simulink model "COMPONENT_MDL_Lag_QUAD_and_PEND_with_Ab"  (R2020b)
settings: Solver=ode23t  StartTime=0.0  StopTime=200  FixedStep=0.001  RelTol=1e-5  EnableMultiTasking=on
undefined symbols (not defined in the file or in its folder): P_pend, P_rot, P_veh_no_props
(part 1 of 12)
settings Model: Creator=bhorton  LastModifiedBy=bhorton
settings DataIOCC: SaveOutput=off  SignalLogging=off  DSMLogging=off  VisualizeSimOutput=off  SaveTime=off  ReturnWorkspaceOutputs=off
settings OptimizationCC: LifeSpan=inf
settings DebuggingCC: AllowSymbolicDim=off  PregeneratedLibrarySubsystemCodeDiagnostic=none  SFUnexpectedBacktrackingDiag=warning  SFNoUnconditionalDefaultTransitionDiag=warning  SFExecutionAtInitializationDiag=none  ArithmeticOperatorsInVariantConditions=warning
settings ModelReferenceCC: PropagateSignalLabelsOutOfModel=off
settings SFSimCC: SimUseLocalCustomCode=off  CustomCodeUndefinedFunction=UseInterfaceOnly
settings RTWCC: RTWUseLocalCustomCode=off
settings CodeAppCC: StateflowObjectComments=on
settings GRTTargetCC: TargetLangStandard=C89/C90 (ANSI)
settings ConfigComp: CovMetricSettings=dw  CovSaveCumulativeToWorkspaceVar=on  CovSaveSingleToWorkspaceVar=on  CovExternalEMLEnable=off
settings SimscapeCC: SimscapeNormalizeSystem=off

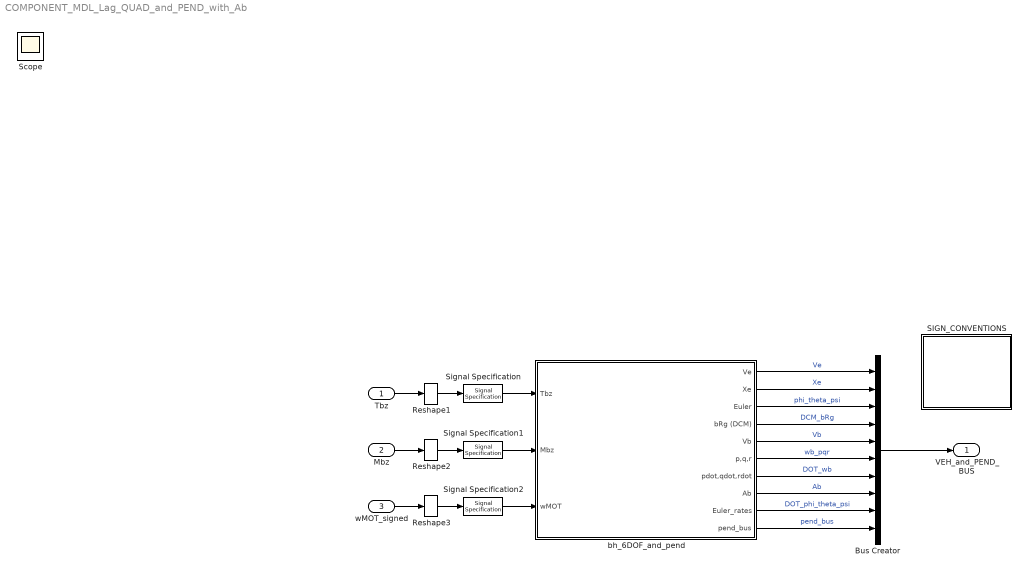
== system COMPONENT_MDL_Lag_QUAD_and_PEND_with_Ab ==
  Tbz : Inport
  Mbz : Inport  Port=2
  wMOT_signed : Inport  Port=3
  Bus Creator : BusCreator  Inputs=10
  Reshape1 : Reshape  OutputDimensionality=Column vector (2-D)
  Reshape2 : Reshape  OutputDimensionality=Column vector (2-D)
  Reshape3 : Reshape  OutputDimensionality=Column vector (2-D)
  SIGN_CONVENTIONS : Subsystem
  Signal Specification : SignalSpecification  Dimensions=[4,1]
  Signal Specification1 : SignalSpecification  Dimensions=[4,1]
  Signal Specification2 : SignalSpecification  Dimensions=[4,1]
  bh_6DOF_and_pend : Subsystem  mask(bh_6DOF EoM (Body Axis)){air_inertia_0=P_veh_no_props.I, air_mass_0=P_veh_no_props.mass, xme_0=P_veh_no_props.Xe_init, Vm_0=P_veh_no_props.Vb_init, pm_0=P_veh_no_props.wb_init, eul_0=P_veh_no_props.eul_init, prop_Imat=P_rot.I, prop_mass=P_rot.mass, prop_CG_L=P_veh_no_props.L_CG_to_mot, prop_CG_H=P_veh_no_props.H_CG_to_mot, g_const=9.80665, I_pend=P_pend.I, m_pend=P_pend.mass, L_pend_XYZ=P_pend.L_xyz, T_pend_XYZ=P_pend.T_xyz, eul_0_pend=P_pend.eul_loc_vec}
      mask prompts: air_inertia_0 "Airframe Inertia, [kg.m^2]"; air_mass_0 "Airframe Mass, [kg]"; xme_0 "Initial position in inertial axes [Xe,Ye,Ze], [m]"; Vm_0 "Initial velocity in body axes [U,v,w], [m/sec]"; pm_0 "Initial body rotation rates [p,q,r], [rad/sec]"; eul_0 "Initial Euler orientation [yaw, pitch, roll], [rad]"; prop_Imat "Propeller Assembly Inertia [kg*m^2]"; prop_mass "Propeller Assembly Mass [kg]"; prop_CG_L "Airframe CG to Prop CG distance - L [m]"; prop_CG_H "Airframe CG to Prop CG distance - H [m]"; g_const "Gravity constant [m/sec^2]"; I_pend "Inertia of Pendulum through it's CoM [kg.m^2]"; m_pend "Mass of pendulum [kg]"; L_pend_XYZ "Lengths of Pendulum (X,Y,Z)  [m]"; T_pend_XYZ "Position of Spherical joint T(X,Y,Z) [m]"; eul_0_pend "Initial Euler orientation [yaw, pitch, roll], [rad]"
      mask DialogControl DescTextVar Prompt: Implementation of a 6-DOF rigid body equations of motion.
      mask DialogControl Control16 Prompt: Euler angles are used to describe angular pose.
      mask DialogControl Container4 Prompt: Airframe
      mask DialogControl Control11 Prompt: ATTENTION:  note the order of the angles in the list above.
      mask DialogControl Control12 Prompt: This is DIFFERENT to the order used in the Aerospace blockset.
      mask DialogControl Container19 Prompt: Propeller
      mask DialogControl Container13 Prompt: ENVIRONMENT
      mask DialogControl Control42 Prompt: NOTE:  the Gravity constant should be a POSITIVE number, eg: 9.81
      mask DialogControl Container14 Prompt: Pendulum
      mask DialogControl Control50 Prompt: Position of Spherical joint relative to airframe CoM:
      mask DialogControl Control41 Prompt: Define the Euler angles of {P}-frame relative to {V}-frame.  The rotation
      mask DialogControl Control45 Prompt: sequence is Z-Y-X  as [Phi,Theta,Psi]
      mask DialogControl Container20 Prompt: Geometry
      mask DialogControl Container21 Prompt: Axes
      mask DialogControl Container6 Prompt: DOC
      mask DialogControl Control6 Prompt: In this EULER angle implementation we define the
      mask DialogControl Control7 Prompt: following sequence that rotates a G-frame
      mask DialogControl Control8 Prompt: into a B-frame:
      mask DialogControl Control9_copy Prompt: 1.)  R1Z  : a local rotation about the Z axis by phi, (YAW)
      mask DialogControl Control9_copy_copy Prompt: 2.)  R2Y  : a local rotation about the Y axis by theta, (PITCH)
      mask DialogControl Control17 Prompt: 3.)  R3X  : a local rotation about the X axis by psi, (ROLL)
      mask DialogControl Container16 Prompt: PASSIVE rotation sequence
      mask DialogControl Control22 Prompt: The co-ordinate transformation that converts the components of a
      mask DialogControl Control23 Prompt: G-frame vector into its components in the B-frame, is:
      mask DialogControl Control24 Prompt: vb = pR3X(psi) * pR2Y(theta) * pR1Z(phi) * vg
      mask DialogControl Control25 Prompt: vb = bRg * vg
      mask DialogControl Control53 Prompt: You can READ more about PASSIVE rotations, HERE.
      mask DialogControl Control53 Callback: winopen('CONCEPT_PASSIVE_rotations.pdf')
      mask DialogControl Container22 Prompt: ACTIVE rotation sequence
      mask DialogControl Control26 Prompt: To actively reposition (ie: rotate) a B-frame that is initially coincident
      mask DialogControl Control27 Prompt: with the inertial G-frame, into a new pose, we would:
      mask DialogControl Control28 Prompt: vg = inv(pR1Z(phi)) * inv(pR2Y(theta)) * inv(pR3X(psi)) * vb
      mask DialogControl Control30 Prompt: If we define:    aR( ) == inv( pR()  ),  then we can write the above as:
      mask DialogControl Control32 Prompt: vg = aR1Z(phi) * aR2Y(theta) * aR3(psi) * vb
      mask DialogControl Control40 Prompt: You can READ more about ACTIVE rotations, HERE.
      mask DialogControl Control40 Callback: winopen('CONCEPT_ACTIVE_rotations.pdf')
      mask Display:
      | port_label('input',1,'{{Tbz_{mot}} (N)}','texmode','on');
      | port_label('input',2,'{{Mbz_{mot}} (N-m)}','texmode','on');
      | port_label('input',3,'{{\omega_{mot}} (rad/sec)}','texmode','on');
      | port_label('output',1,'{V_e (m/s)}','texmode','on');
      | port_label('output',2,'{X_e (m)}','texmode','on');
      | port_label('output',3,'{\Phi_{Z1} \theta_{Y2} \Psi_{X3} (rad)}','texmode','on');
      | port_label('output',4,'{DCM bRg }','texmode','on');
      | port_label('output',5,'{V_b (m/s)}','texmode','on');
      | port_label('output',6,'{{\omega_b (rad/s)}}','texmode','on');
      | port_label('output',7,'{{d\omega_b/dt}}','texmode','on');
      | port_label('output',8,'{A_b (m/s^2)}','texmode','on');
      | port_label('output',9,'{d\Phi_{Z1} d\theta_{Y2} d\Psi_{X3} (rad/sec)}','texmode','on');
      | 
      | %text(0.5,0.7248,'Simscape \nBody\nEuler Angles \n\n\n\n\n PENDULUM','horizontalAlignment','center')
      | %text(0.5,0.3112,'Fixed\nMass','horizontalAlignment','center')
      | %image(imread('bh_LAG_EQN.JPG'),[0.27, 0.25,0.5,0.35])
      | 
      | text(0.5,0.7248,'Quad\n+ PENDULUM','horizontalAlignment','center')
      | %text(0.5,0.3112,'Fixed\nMass','horizontalAlignment','center')
      | image(imread('bh_LAG_EQN.JPG'),[0.27, 0.25,0.5,0.35])
  VEH_and_PEND_BUS : Outport  OutDataTypeStr=Bus: VEH_AND_PEND_BUS  VectorParamsAs1DForOutWhenUnconnected=off
  Scope : Scope
  wires:
  wMOT_signed/1 -> Reshape3/1
  Tbz/1 -> Reshape1/1
  bh_6DOF_and_pend/6(p,q,r) -> Bus Creator/6  "wb_pqr"
  Bus Creator/1 -> VEH_and_PEND_BUS/1
  bh_6DOF_and_pend/7(pdot,qdot,rdot) -> Bus Creator/7  "DOT_wb"
  Reshape1/1 -> Signal Specification/1
  bh_6DOF_and_pend/1(Ve) -> Bus Creator/1  "Ve"
  Signal Specification2/1 -> bh_6DOF_and_pend/3(wMOT)
  Signal Specification/1 -> bh_6DOF_and_pend/1(Tbz)
  bh_6DOF_and_pend/9(Euler_rates) -> Bus Creator/9  "DOT_phi_theta_psi"
  bh_6DOF_and_pend/2(Xe) -> Bus Creator/2  "Xe"
  bh_6DOF_and_pend/8(Ab) -> Bus Creator/8  "Ab"
  Reshape3/1 -> Signal Specification2/1
  Reshape2/1 -> Signal Specification1/1
  bh_6DOF_and_pend/3(Euler) -> Bus Creator/3  "phi_theta_psi"
  Signal Specification1/1 -> bh_6DOF_and_pend/2(Mbz)
  bh_6DOF_and_pend/4(bRg (DCM)) -> Bus Creator/4  "DCM_bRg"
  bh_6DOF_and_pend/5(Vb) -> Bus Creator/5  "Vb"
  Mbz/1 -> Reshape2/1
  bh_6DOF_and_pend/10(pend_bus) -> Bus Creator/10  "pend_bus"

== system COMPONENT_MDL_Lag_QUAD_and_PEND_with_Ab/SIGN_CONVENTIONS ==

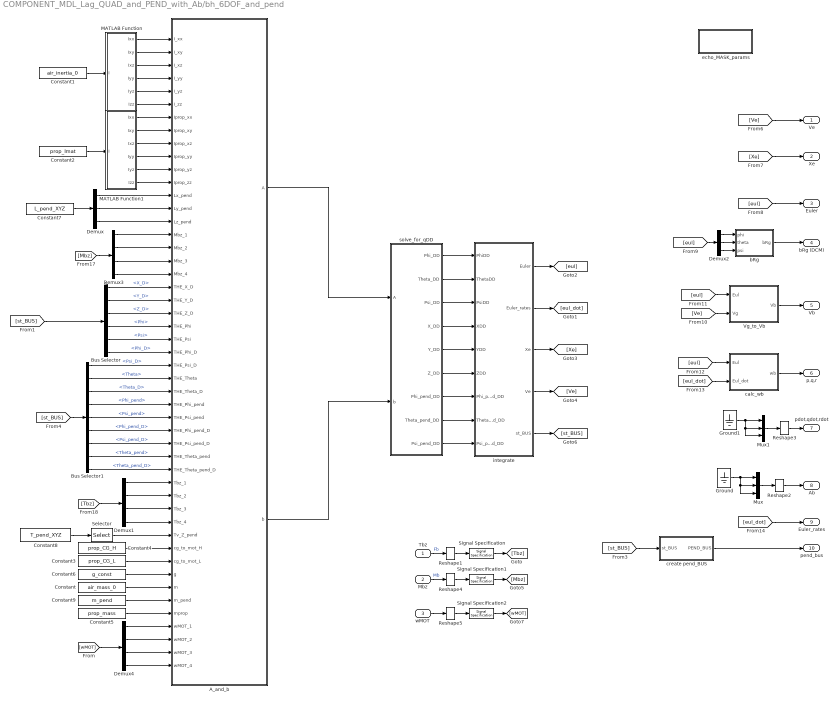
== system COMPONENT_MDL_Lag_QUAD_and_PEND_with_Ab/bh_6DOF_and_pend ==
  Tbz : Inport
  Mbz : Inport  Port=2
  wMOT : Inport  Port=3
  A_and_b : MATLAB Function  TreatAsAtomicUnit=on
  Bus Selector : BusSelector  OutputSignals=Vel_list.X_D,Vel_list.Y_D,Vel_list.Z_D,Pos_list.Phi,Pos_list.Psi,Vel_list.Phi_D
  Bus Selector1 : BusSelector  OutputSignals=Vel_list.Psi_D,Pos_list.Theta,Vel_list.Theta_D,Pos_list.Phi_pend,Pos_list.Psi_pend,Vel_list.Phi_pend_D,Vel_list.Psi_pend_D,Pos_list.Theta_pend,Vel_list.Theta_pend_D
  Constant : Constant  Value=air_mass_0  OutDataTypeStr=Inherit: Inherit via back propagation
  Constant1 : Constant  Value=air_inertia_0  OutDataTypeStr=Inherit: Inherit via back propagation
  Constant2 : Constant  Value=prop_Imat  OutDataTypeStr=Inherit: Inherit via back propagation
  Constant3 : Constant  Value=prop_CG_L  OutDataTypeStr=Inherit: Inherit via back propagation
  Constant4 : Constant  Value=prop_CG_H  OutDataTypeStr=Inherit: Inherit via back propagation
  Constant5 : Constant  Value=prop_mass  OutDataTypeStr=Inherit: Inherit via back propagation
  Constant6 : Constant  Value=g_const  OutDataTypeStr=Inherit: Inherit via back propagation
  Constant7 : Constant  Value=L_pend_XYZ  OutDataTypeStr=Inherit: Inherit via back propagation
  Constant8 : Constant  Value=T_pend_XYZ
  Constant9 : Constant  Value=m_pend  OutDataTypeStr=Inherit: Inherit via back propagation
  Demux : Demux  Outputs=3
  Demux1 : Demux
  Demux2 : Demux  Outputs=3
  Demux3 : Demux
  Demux4 : Demux
  Ground : Ground
  Ground1 : Ground
  MATLAB Function : MATLAB Function  TreatAsAtomicUnit=on
  MATLAB Function1 : MATLAB Function  TreatAsAtomicUnit=on
  Mux : Mux  Inputs=3
  Mux1 : Mux  Inputs=3
  Reshape{1..5} (5 alike) : Reshape  OutputDimensionality=Column vector (2-D)
  Selector : Selector  InputPortWidth=3  IndexOptions=Index vector (dialog)  Indices=3  OutputSizes=1
  Signal Specification : SignalSpecification  Dimensions=[4,1]
  Signal Specification1 : SignalSpecification  Dimensions=[4,1]
  Signal Specification2 : SignalSpecification  Dimensions=[4,1]
  Vg_to_Vb : Subsystem
  bRg : MATLAB Function  TreatAsAtomicUnit=on
  calc_wb : Subsystem
  create pend_BUS : Subsystem
  echo_MASK_params : Subsystem
  integrate : Subsystem
  solve_for_qDD : Subsystem
  Ve : Outport  VectorParamsAs1DForOutWhenUnconnected=off
  Xe : Outport  Port=2  VectorParamsAs1DForOutWhenUnconnected=off
  Euler : Outport  Port=3  VectorParamsAs1DForOutWhenUnconnected=off
  bRg (DCM) : Outport  Port=4  VectorParamsAs1DForOutWhenUnconnected=off
  Vb : Outport  Port=5  VectorParamsAs1DForOutWhenUnconnected=off
  p,q,r : Outport  Port=6  VectorParamsAs1DForOutWhenUnconnected=off
  pdot,qdot,rdot : Outport  Port=7  VectorParamsAs1DForOutWhenUnconnected=off
  Ab : Outport  Port=8  VectorParamsAs1DForOutWhenUnconnected=off
  Euler_rates : Outport  Port=9  VectorParamsAs1DForOutWhenUnconnected=off
  pend_bus : Outport  Port=10  VectorParamsAs1DForOutWhenUnconnected=off
  wires:
  Mux1/1 -> Reshape3/1
  MATLAB Function/5(Iyz) -> A_and_b/5(I_yz)
  Demux2/1 -> bRg/1(phi)
  Demux4/3 -> A_and_b/48(wMOT_3)
  Demux3/1 -> A_and_b/16(Mbz_1)
  [Xe] -> Xe/1
  MATLAB Function1/6(Izz) -> A_and_b/12(Iprop_zz)
  Tbz/1 -> Reshape1/1  "Fb"
  integrate/5(st_BUS) -> [st_BUS]
  Constant5/1 -> A_and_b/45(mprop)
  [Ve] -> Ve/1
  Ground/1 -> Mux/2, Mux/3, Mux/1
  Reshape3/1 -> pdot,qdot,rdot/1
  MATLAB Function1/2(Ixy) -> A_and_b/8(Iprop_xy)
  MATLAB Function/3(Ixz) -> A_and_b/3(I_xz)
  calc_wb/1(wb) -> p,q,r/1
  integrate/4(Ve) -> [Ve]
  Demux4/2 -> A_and_b/47(wMOT_2)
  Demux3/2 -> A_and_b/17(Mbz_2)
  [eul] -> Vg_to_Vb/1(Eul)
  Demux1/2 -> A_and_b/36(Tbz_2)
  [st_BUS] -> Bus Selector/1
  [Ve] -> Vg_to_Vb/2(Vg)
  Reshape4/1 -> Signal Specification1/1
  Demux1/1 -> A_and_b/35(Tbz_1)
  [eul] -> calc_wb/1(Eul)
  solve_for_qDD/5(Y_DD) -> integrate/5(YDD)
  MATLAB Function1/3(Ixz) -> A_and_b/9(Iprop_xz)
  Demux3/4 -> A_and_b/19(Mbz_4)
  integrate/1(Euler) -> [eul]
  [eul_dot] -> Euler_rates/1
  Demux2/3 -> bRg/3(psi)
  Constant/1 -> A_and_b/43(m)
  solve_for_qDD/6(Z_DD) -> integrate/6(ZDD)
  [Tbz] -> Demux1/1
  Mux/1 -> Reshape2/1
  solve_for_qDD/3(Psi_DD) -> integrate/3(PsiDD)
  Demux1/4 -> A_and_b/38(Tbz_4)
  MATLAB Function/2(Ixy) -> A_and_b/2(I_xy)
  Signal Specification/1 -> [Tbz]
  [eul_dot] -> calc_wb/2(Eul_dot)
  Demux4/1 -> A_and_b/46(wMOT_1)
  Reshape5/1 -> Signal Specification2/1
  wMOT/1 -> Reshape5/1
  Signal Specification1/1 -> [Mbz]
  solve_for_qDD/1(Phi_DD) -> integrate/1(PhiDD)
  MATLAB Function1/5(Iyz) -> A_and_b/11(Iprop_yz)
  MATLAB Function1/4(Iyy) -> A_and_b/10(Iprop_yy)
  Ground1/1 -> Mux1/2, Mux1/3, Mux1/1
  [eul] -> Demux2/1
  solve_for_qDD/2(Theta_DD) -> integrate/2(ThetaDD)
  MATLAB Function/6(Izz) -> A_and_b/6(I_zz)
  Reshape1/1 -> Signal Specification/1
  [eul] -> Euler/1
  Signal Specification2/1 -> [wMOT]
  MATLAB Function1/1(Ixx) -> A_and_b/7(Iprop_xx)
  [Mbz] -> Demux3/1
  Demux3/3 -> A_and_b/18(Mbz_3)
  Vg_to_Vb/1(Vb) -> Vb/1
  Reshape2/1 -> Ab/1
  Constant2/1 -> MATLAB Function1/1(I)
  integrate/3(Xe) -> [Xe]
  Mbz/1 -> Reshape4/1  "Mb"
  integrate/2(Euler_rates) -> [eul_dot]
  Demux1/3 -> A_and_b/37(Tbz_3)
  MATLAB Function/4(Iyy) -> A_and_b/4(I_yy)
  Demux2/2 -> bRg/2(theta)
  Constant4/1 -> A_and_b/40(cg_to_mot_H)
  solve_for_qDD/4(X_DD) -> integrate/4(XDD)
  [wMOT] -> Demux4/1
  Constant6/1 -> A_and_b/42(g)
  MATLAB Function/1(Ixx) -> A_and_b/1(I_xx)
  Constant1/1 -> MATLAB Function/1(I)
  bRg/1(bRg) -> bRg (DCM)/1
  Constant3/1 -> A_and_b/41(cg_to_mot_L)
  create pend_BUS/1(PEND_BUS) -> pend_bus/1
  Demux/3 -> A_and_b/15(Lz_pend)
  Demux/2 -> A_and_b/14(Ly_pend)
  Demux/1 -> A_and_b/13(Lx_pend)
  Constant7/1 -> Demux/1
  Constant8/1 -> Selector/1
  Selector/1 -> A_and_b/39(Tv_Z_pend)
  Constant9/1 -> A_and_b/44(m_pend)
  solve_for_qDD/7(Phi_pend_DD) -> integrate/7(Phi_pend_DD)
  solve_for_qDD/8(Theta_pend_DD) -> integrate/8(Theta_pend_DD)
  solve_for_qDD/9(Psi_pend_DD) -> integrate/9(Psi_pend_DD)
  [st_BUS] -> create pend_BUS/1(st_BUS)
  [st_BUS] -> Bus Selector1/1
  Demux4/4 -> A_and_b/49(wMOT_4)
  Bus Selector/1 -> A_and_b/20(THE_X_D)  "<X_D>"
  Bus Selector/2 -> A_and_b/21(THE_Y_D)  "<Y_D>"
  Bus Selector/3 -> A_and_b/22(THE_Z_D)  "<Z_D>"
  Bus Selector/4 -> A_and_b/23(THE_Phi)  "<Phi>"
  Bus Selector/5 -> A_and_b/24(THE_Psi)  "<Psi>"
  Bus Selector/6 -> A_and_b/25(THE_Phi_D)  "<Phi_D>"
  Bus Selector1/3 -> A_and_b/28(THE_Theta_D)  "<Theta_D>"
  Bus Selector1/2 -> A_and_b/27(THE_Theta)  "<Theta>"
  Bus Selector1/4 -> A_and_b/29(THE_Phi_pend)  "<Phi_pend>"
  Bus Selector1/1 -> A_and_b/26(THE_Psi_D)  "<Psi_D>"
  Bus Selector1/5 -> A_and_b/30(THE_Psi_pend)  "<Psi_pend>"
  Bus Selector1/6 -> A_and_b/31(THE_Phi_pend_D)  "<Phi_pend_D>"
  Bus Selector1/7 -> A_and_b/32(THE_Psi_pend_D)  "<Psi_pend_D>"
  Bus Selector1/8 -> A_and_b/33(THE_Theta_pend)  "<Theta_pend>"
  Bus Selector1/9 -> A_and_b/34(THE_Theta_pend_D)  "<Theta_pend_D>"
  A_and_b/1(A) -> solve_for_qDD/1(A)
  A_and_b/2(b) -> solve_for_qDD/2(b)

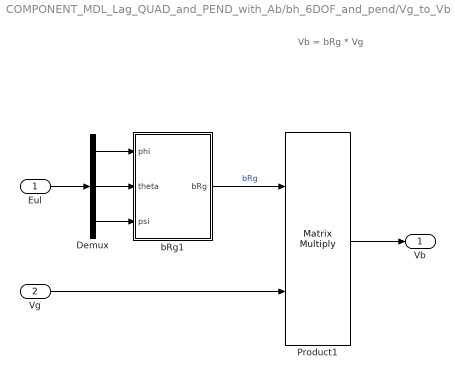
== system COMPONENT_MDL_Lag_QUAD_and_PEND_with_Ab/bh_6DOF_and_pend/Vg_to_Vb ==
  note: Vb = bRg * Vg
  Eul : Inport
  Vg : Inport  Port=2
  Demux : Demux  Outputs=3
  Product1 : Product  Multiplication=Matrix(*)  InputSameDT=on  SaturateOnIntegerOverflow=on  OutDataTypeStr=Inherit: Same as first input
  bRg1 : MATLAB Function  TreatAsAtomicUnit=on
  Vb : Outport  VectorParamsAs1DForOutWhenUnconnected=off
  wires:
  bRg1/1(bRg) -> Product1/1  "bRg"
  Demux/1 -> bRg1/1(phi)
  Demux/2 -> bRg1/2(theta)
  Demux/3 -> bRg1/3(psi)
  Eul/1 -> Demux/1
  Product1/1 -> Vb/1
  Vg/1 -> Product1/2

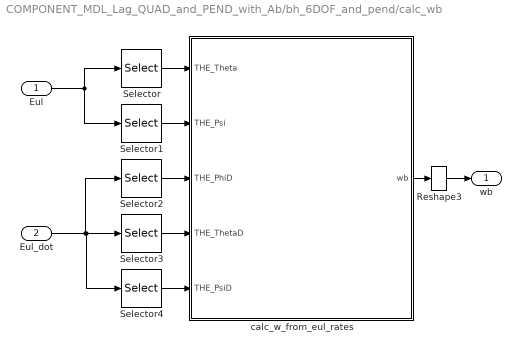
== system COMPONENT_MDL_Lag_QUAD_and_PEND_with_Ab/bh_6DOF_and_pend/calc_wb ==
  Eul : Inport
  Eul_dot : Inport  Port=2
  Reshape3 : Reshape  OutputDimensionality=Column vector (2-D)
  Selector : Selector  InputPortWidth=3  IndexOptions=Index vector (dialog)  Indices=2  OutputSizes=1
  Selector1 : Selector  InputPortWidth=3  IndexOptions=Index vector (dialog)  Indices=3  OutputSizes=1
  Selector2 : Selector  InputPortWidth=3  IndexOptions=Index vector (dialog)  Indices=1  OutputSizes=1
  Selector3 : Selector  InputPortWidth=3  IndexOptions=Index vector (dialog)  Indices=2  OutputSizes=1
  Selector4 : Selector  InputPortWidth=3  IndexOptions=Index vector (dialog)  Indices=3  OutputSizes=1
  calc_w_from_eul_rates : MATLAB Function  TreatAsAtomicUnit=on
  wb : Outport  VectorParamsAs1DForOutWhenUnconnected=off
  wires:
  calc_w_from_eul_rates/1(wb) -> Reshape3/1
  Eul/1 -> Selector/1, Selector1/1
  Selector/1 -> calc_w_from_eul_rates/1(THE_Theta)
  Selector1/1 -> calc_w_from_eul_rates/2(THE_Psi)
  Selector2/1 -> calc_w_from_eul_rates/3(THE_PhiD)
  Eul_dot/1 -> Selector2/1, Selector4/1, Selector3/1
  Selector3/1 -> calc_w_from_eul_rates/4(THE_ThetaD)
  Selector4/1 -> calc_w_from_eul_rates/5(THE_PsiD)
  Reshape3/1 -> wb/1

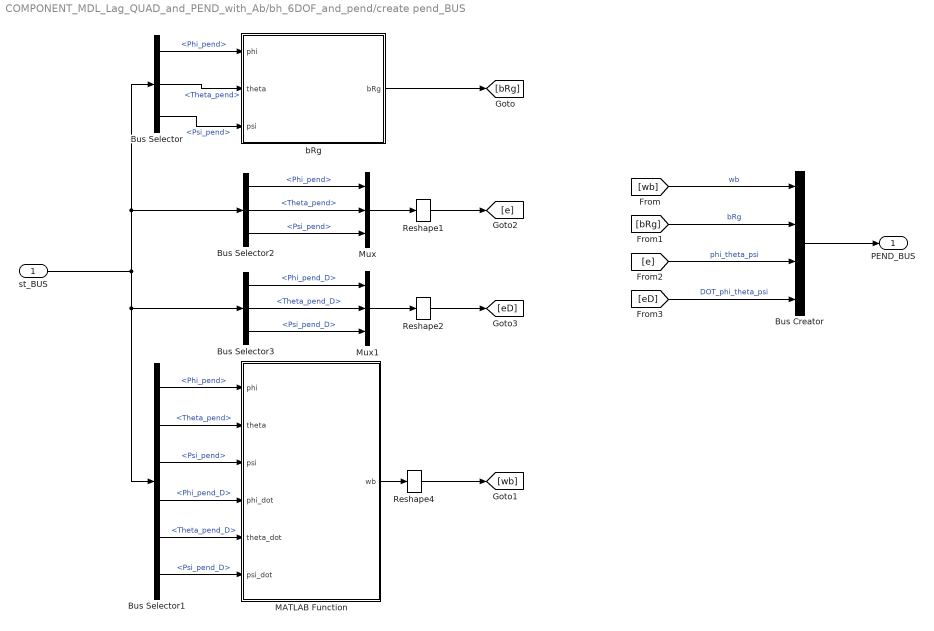
== system COMPONENT_MDL_Lag_QUAD_and_PEND_with_Ab/bh_6DOF_and_pend/create pend_BUS ==
  st_BUS : Inport
  Bus Creator : BusCreator  Inputs=4
  Bus Selector : BusSelector  OutputSignals=Pos_list.Phi_pend,Pos_list.Theta_pend,Pos_list.Psi_pend
  Bus Selector1 : BusSelector  OutputSignals=Pos_list.Phi_pend,Pos_list.Theta_pend,Pos_list.Psi_pend,Vel_list.Phi_pend_D,Vel_list.Theta_pend_D,Vel_list.Psi_pend_D
  Bus Selector2 : BusSelector  OutputSignals=Pos_list.Phi_pend,Pos_list.Theta_pend,Pos_list.Psi_pend
  Bus Selector3 : BusSelector  OutputSignals=Vel_list.Phi_pend_D,Vel_list.Theta_pend_D,Vel_list.Psi_pend_D
  MATLAB Function : MATLAB Function  TreatAsAtomicUnit=on
  Mux : Mux  Inputs=3
  Mux1 : Mux  Inputs=3
  Reshape1 : Reshape  OutputDimensionality=Column vector (2-D)
  Reshape2 : Reshape  OutputDimensionality=Column vector (2-D)
  Reshape4 : Reshape  OutputDimensionality=Column vector (2-D)
  bRg : MATLAB Function  TreatAsAtomicUnit=on
  PEND_BUS : Outport  VectorParamsAs1DForOutWhenUnconnected=off
  wires:
  [eD] -> Bus Creator/4  "DOT_phi_theta_psi"
  Bus Creator/1 -> PEND_BUS/1
  [e] -> Bus Creator/3  "phi_theta_psi"
  [bRg] -> Bus Creator/2  "bRg"
  [wb] -> Bus Creator/1  "wb"
  bRg/1(bRg) -> [bRg]
  st_BUS/1 -> Bus Selector/1, Bus Selector2/1, Bus Selector3/1, Bus Selector1/1
  Bus Selector/1 -> bRg/1(phi)  "<Phi_pend>"
  Bus Selector/2 -> bRg/2(theta)  "<Theta_pend>"
  Bus Selector/3 -> bRg/3(psi)  "<Psi_pend>"
  Bus Selector1/1 -> MATLAB Function/1(phi)  "<Phi_pend>"
  Bus Selector1/2 -> MATLAB Function/2(theta)  "<Theta_pend>"
  Bus Selector1/3 -> MATLAB Function/3(psi)  "<Psi_pend>"
  Bus Selector1/4 -> MATLAB Function/4(phi_dot)  "<Phi_pend_D>"
  Bus Selector1/5 -> MATLAB Function/5(theta_dot)  "<Theta_pend_D>"
  Bus Selector1/6 -> MATLAB Function/6(psi_dot)  "<Psi_pend_D>"
  MATLAB Function/1(wb) -> Reshape4/1
  Reshape4/1 -> [wb]
  Bus Selector2/1 -> Mux/1  "<Phi_pend>"
  Bus Selector2/2 -> Mux/2  "<Theta_pend>"
  Bus Selector2/3 -> Mux/3  "<Psi_pend>"
  Bus Selector3/1 -> Mux1/1  "<Phi_pend_D>"
  Bus Selector3/2 -> Mux1/2  "<Theta_pend_D>"
  Bus Selector3/3 -> Mux1/3  "<Psi_pend_D>"
  Mux/1 -> Reshape1/1
  Mux1/1 -> Reshape2/1
  Reshape2/1 -> [eD]
  Reshape1/1 -> [e]

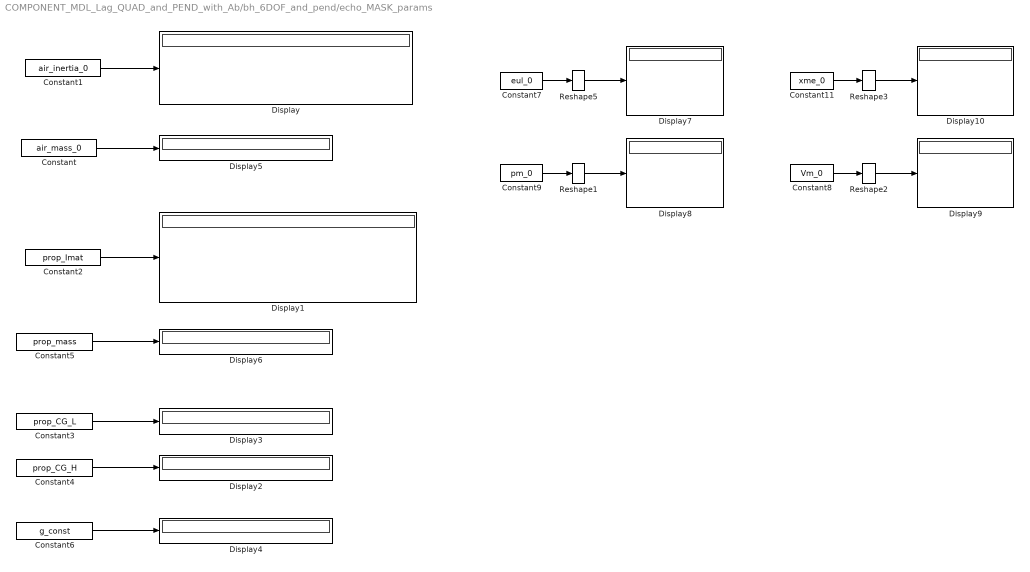
== system COMPONENT_MDL_Lag_QUAD_and_PEND_with_Ab/bh_6DOF_and_pend/echo_MASK_params ==
  Constant : Constant  Value=air_mass_0  OutDataTypeStr=Inherit: Inherit via back propagation
  Constant1 : Constant  Value=air_inertia_0  OutDataTypeStr=Inherit: Inherit via back propagation
  Constant11 : Constant  Value=xme_0  OutDataTypeStr=Inherit: Inherit via back propagation
  Constant2 : Constant  Value=prop_Imat  OutDataTypeStr=Inherit: Inherit via back propagation
  Constant3 : Constant  Value=prop_CG_L  OutDataTypeStr=Inherit: Inherit via back propagation
  Constant4 : Constant  Value=prop_CG_H  OutDataTypeStr=Inherit: Inherit via back propagation
  Constant5 : Constant  Value=prop_mass  OutDataTypeStr=Inherit: Inherit via back propagation
  Constant6 : Constant  Value=g_const  OutDataTypeStr=Inherit: Inherit via back propagation
  Constant7 : Constant  Value=eul_0  OutDataTypeStr=Inherit: Inherit via back propagation
  Constant8 : Constant  Value=Vm_0  OutDataTypeStr=Inherit: Inherit via back propagation
  Constant9 : Constant  Value=pm_0  OutDataTypeStr=Inherit: Inherit via back propagation
  Display{,1..10} (11 alike) : Display
  Reshape{1..3,5} (4 alike) : Reshape  OutputDimensionality=Column vector (2-D)
  wires:
  Constant2/1 -> Display1/1
  Constant1/1 -> Display/1
  Constant4/1 -> Display2/1
  Constant6/1 -> Display4/1
  Constant/1 -> Display5/1
  Constant5/1 -> Display6/1
  Constant3/1 -> Display3/1
  Constant7/1 -> Reshape5/1
  Reshape5/1 -> Display7/1
  Reshape1/1 -> Display8/1
  Constant9/1 -> Reshape1/1
  Reshape2/1 -> Display9/1
  Constant8/1 -> Reshape2/1
  Reshape3/1 -> Display10/1
  Constant11/1 -> Reshape3/1

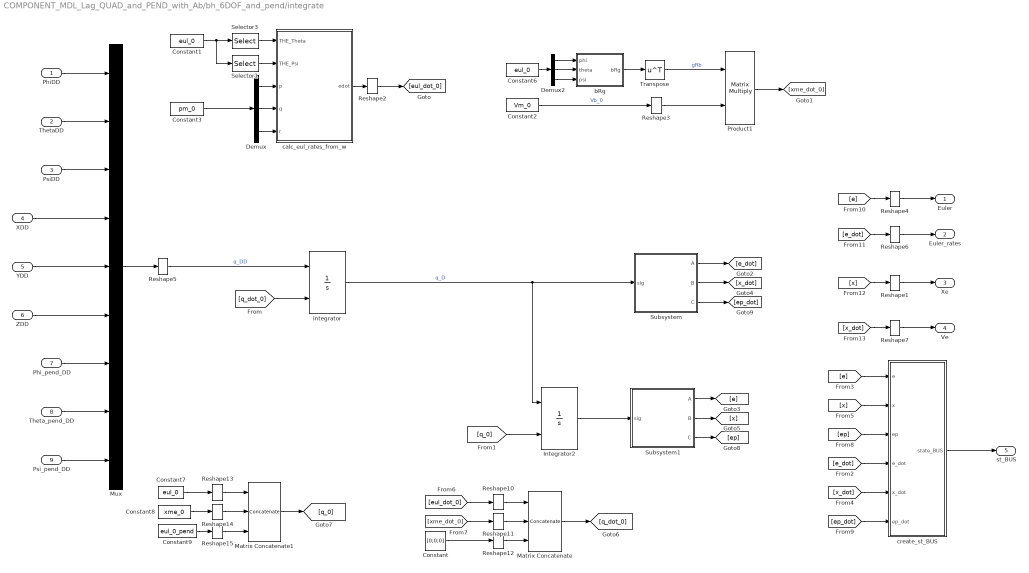
== system COMPONENT_MDL_Lag_QUAD_and_PEND_with_Ab/bh_6DOF_and_pend/integrate ==
  PhiDD : Inport
  ThetaDD : Inport  Port=2
  PsiDD : Inport  Port=3
  XDD : Inport  Port=4
  YDD : Inport  Port=5
  ZDD : Inport  Port=6
  Phi_pend_DD : Inport  Port=7
  Theta_pend_DD : Inport  Port=8
  Psi_pend_DD : Inport  Port=9
  Constant : Constant  Value=[0;0;0]  VectorParams1D=off
  Constant1 : Constant  Value=eul_0  OutDataTypeStr=Inherit: Inherit via back propagation
  Constant2 : Constant  Value=Vm_0  OutDataTypeStr=Inherit: Inherit via back propagation
  Constant3 : Constant  Value=pm_0  OutDataTypeStr=Inherit: Inherit via back propagation
  Constant6 : Constant  Value=eul_0  OutDataTypeStr=Inherit: Inherit via back propagation
  Constant7 : Constant  Value=eul_0  OutDataTypeStr=Inherit: Inherit via back propagation
  Constant8 : Constant  Value=xme_0  OutDataTypeStr=Inherit: Inherit via back propagation
  Constant9 : Constant  Value=eul_0_pend  OutDataTypeStr=Inherit: Inherit via back propagation
  Demux : Demux  Outputs=3
  Demux2 : Demux  Outputs=3
  Integrator : Integrator  InitialConditionSource=external  ContinuousStateAttributes={'DOT_phi', 'DOT_theta','DOT_psi','DOT_Xe', 'DOT_Ye', 'DOT_Ze','DOT_phi_pend', 'DOT_theta_pend','DOT_psi_pend'}
      settings: AttributesFormatString=%<ContinuousStateAttributes>
  Integrator2 : Integrator  InitialConditionSource=external  ContinuousStateAttributes="{'phi', 'theta','psi','Xe', 'Ye', 'Ze',  'phi_pend', 'theta_pend','psi_pend'}"
      settings: AttributesFormatString=%<ContinuousStateAttributes>
  Matrix Concatenate : Concatenate  NumInputs=3  Mode=Multidimensional array
  Matrix Concatenate1 : Concatenate  NumInputs=3  Mode=Multidimensional array
  Mux : Mux  Inputs=9
  Product1 : Product  Multiplication=Matrix(*)  InputSameDT=on  SaturateOnIntegerOverflow=on  OutDataTypeStr=Inherit: Same as first input
  Reshape{1..7,10..15} (13 alike) : Reshape  OutputDimensionality=Column vector (2-D)
  Selector1 : Selector  InputPortWidth=3  IndexOptions=Index vector (dialog)  Indices=3  OutputSizes=1
  Selector3 : Selector  InputPortWidth=3  IndexOptions=Index vector (dialog)  Indices=2  OutputSizes=1
  Subsystem : Subsystem
  Subsystem1 : Subsystem
  Transpose : Math  Operator=transpose  SignedPower=on  SaturateOnIntegerOverflow=on
  bRg : MATLAB Function  TreatAsAtomicUnit=on
  calc_eul_rates_from_w : MATLAB Function  TreatAsAtomicUnit=on
  create_st_BUS : Subsystem
  Euler : Outport  VectorParamsAs1DForOutWhenUnconnected=off
  Euler_rates : Outport  Port=2  VectorParamsAs1DForOutWhenUnconnected=off
  Xe : Outport  Port=3  VectorParamsAs1DForOutWhenUnconnected=off
  Ve : Outport  Port=4  VectorParamsAs1DForOutWhenUnconnected=off
  st_BUS : Outport  Port=5  VectorParamsAs1DForOutWhenUnconnected=off
  wires:
  PhiDD/1 -> Mux/1
  ThetaDD/1 -> Mux/2
  PsiDD/1 -> Mux/3
  Mux/1 -> Reshape5/1
  Integrator/1 -> Subsystem/1(sig), Integrator2/1  "q_D"
  Reshape5/1 -> Integrator/1  "q_DD"
  [q_0] -> Integrator2/2
  Constant1/1 -> Selector1/1, Selector3/1
  [q_dot_0] -> Integrator/2
  Constant2/1 -> Reshape3/1  "Vb_0"
  bRg/1(bRg) -> Transpose/1
  Reshape3/1 -> Product1/2
  Constant6/1 -> Demux2/1
  Transpose/1 -> Product1/1  "gRb"
  Product1/1 -> [xme_dot_0]
  Reshape4/1 -> Euler/1
  Reshape6/1 -> Euler_rates/1
  Reshape1/1 -> Xe/1
  Reshape7/1 -> Ve/1
  Demux2/1 -> bRg/1(phi)
  Demux2/2 -> bRg/2(theta)
  Demux2/3 -> bRg/3(psi)
  Selector3/1 -> calc_eul_rates_from_w/1(THE_Theta)
  Selector1/1 -> calc_eul_rates_from_w/2(THE_Psi)
  Demux/3 -> calc_eul_rates_from_w/5(r)
  Demux/2 -> calc_eul_rates_from_w/4(q)
  Demux/1 -> calc_eul_rates_from_w/3(p)
  calc_eul_rates_from_w/1(edot) -> Reshape2/1
  Constant3/1 -> Demux/1
  Reshape2/1 -> [eul_dot_0]
  create_st_BUS/1(state_BUS) -> st_BUS/1
  [eul_dot_0] -> Reshape10/1
  [xme_dot_0] -> Reshape11/1
  Constant/1 -> Reshape12/1
  Reshape12/1 -> Matrix Concatenate/3
  Reshape11/1 -> Matrix Concatenate/2
  Reshape10/1 -> Matrix Concatenate/1
  Constant8/1 -> Reshape14/1
  Reshape15/1 -> Matrix Concatenate1/3
  Reshape13/1 -> Matrix Concatenate1/1
  Constant7/1 -> Reshape13/1
  Reshape14/1 -> Matrix Concatenate1/2
  Constant9/1 -> Reshape15/1
  YDD/1 -> Mux/5
  ZDD/1 -> Mux/6
  XDD/1 -> Mux/4
  Psi_pend_DD/1 -> Mux/9
  Theta_pend_DD/1 -> Mux/8
  Phi_pend_DD/1 -> Mux/7
  Matrix Concatenate/1 -> [q_dot_0]
  Matrix Concatenate1/1 -> [q_0]
  Integrator2/1 -> Subsystem1/1(sig)
  Subsystem1/3(C) -> [ep]
  Subsystem1/2(B) -> [x]
  Subsystem1/1(A) -> [e]
  Subsystem/1(A) -> [e_dot]
  Subsystem/2(B) -> [x_dot]
  Subsystem/3(C) -> [ep_dot]
  [e] -> Reshape4/1
  [e_dot] -> Reshape6/1
  [x] -> Reshape1/1
  [x_dot] -> Reshape7/1
  [e] -> create_st_BUS/1(e)
  [x] -> create_st_BUS/2(x)
  [ep] -> create_st_BUS/3(ep)
  [e_dot] -> create_st_BUS/4(e_dot)
  [x_dot] -> create_st_BUS/5(x_dot)
  [ep_dot] -> create_st_BUS/6(ep_dot)

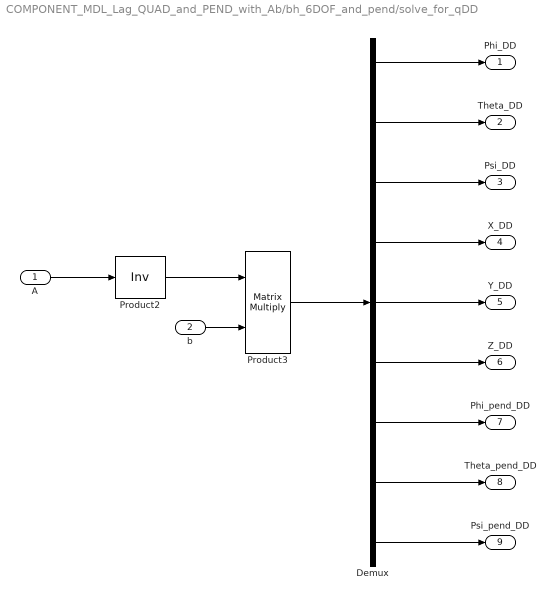
== system COMPONENT_MDL_Lag_QUAD_and_PEND_with_Ab/bh_6DOF_and_pend/solve_for_qDD ==
  A : Inport
  b : Inport  Port=2
  Demux : Demux  Outputs=9
  Product2 : Product  Inputs=/  Multiplication=Matrix(*)
  Product3 : Product  Multiplication=Matrix(*)
  Phi_DD : Outport  VectorParamsAs1DForOutWhenUnconnected=off
  Theta_DD : Outport  Port=2  VectorParamsAs1DForOutWhenUnconnected=off
  Psi_DD : Outport  Port=3  VectorParamsAs1DForOutWhenUnconnected=off
  X_DD : Outport  Port=4  VectorParamsAs1DForOutWhenUnconnected=off
  Y_DD : Outport  Port=5  VectorParamsAs1DForOutWhenUnconnected=off
  Z_DD : Outport  Port=6  VectorParamsAs1DForOutWhenUnconnected=off
  Phi_pend_DD : Outport  Port=7  VectorParamsAs1DForOutWhenUnconnected=off
  Theta_pend_DD : Outport  Port=8  VectorParamsAs1DForOutWhenUnconnected=off
  Psi_pend_DD : Outport  Port=9  VectorParamsAs1DForOutWhenUnconnected=off
  wires:
  A/1 -> Product2/1
  Product2/1 -> Product3/1
  Product3/1 -> Demux/1
  Demux/1 -> Phi_DD/1
  Demux/2 -> Theta_DD/1
  Demux/3 -> Psi_DD/1
  Demux/4 -> X_DD/1
  Demux/6 -> Z_DD/1
  Demux/5 -> Y_DD/1
  Demux/9 -> Psi_pend_DD/1
  Demux/8 -> Theta_pend_DD/1
  Demux/7 -> Phi_pend_DD/1
  b/1 -> Product3/2

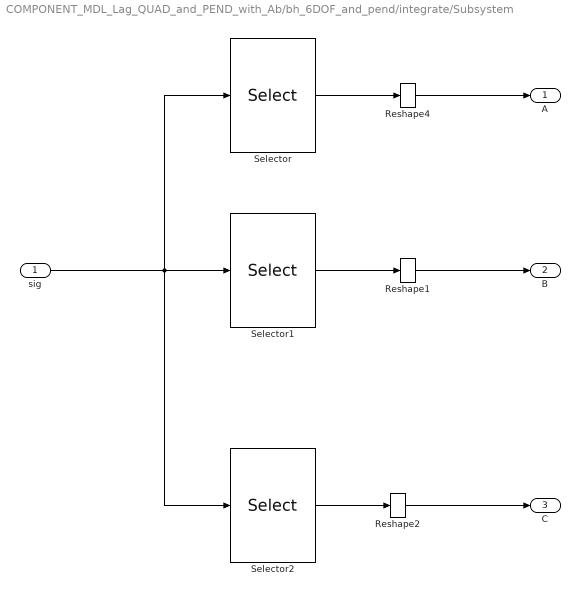
== system COMPONENT_MDL_Lag_QUAD_and_PEND_with_Ab/bh_6DOF_and_pend/integrate/Subsystem ==
  sig : Inport
  Reshape1 : Reshape  OutputDimensionality=Column vector (2-D)
  Reshape2 : Reshape  OutputDimensionality=Column vector (2-D)
  Reshape4 : Reshape  OutputDimensionality=Column vector (2-D)
  Selector : Selector  InputPortWidth=9  IndexOptions=Index vector (dialog)  Indices=1:3  OutputSizes=1
  Selector1 : Selector  InputPortWidth=9  IndexOptions=Index vector (dialog)  Indices=4:6  OutputSizes=1
  Selector2 : Selector  InputPortWidth=9  IndexOptions=Index vector (dialog)  Indices=7:9  OutputSizes=1
  A : Outport  VectorParamsAs1DForOutWhenUnconnected=off
  B : Outport  Port=2  VectorParamsAs1DForOutWhenUnconnected=off
  C : Outport  Port=3  VectorParamsAs1DForOutWhenUnconnected=off
  wires:
  Selector/1 -> Reshape4/1
  Selector2/1 -> Reshape2/1
  Selector1/1 -> Reshape1/1
  sig/1 -> Selector/1, Selector2/1, Selector1/1
  Reshape4/1 -> A/1
  Reshape1/1 -> B/1
  Reshape2/1 -> C/1

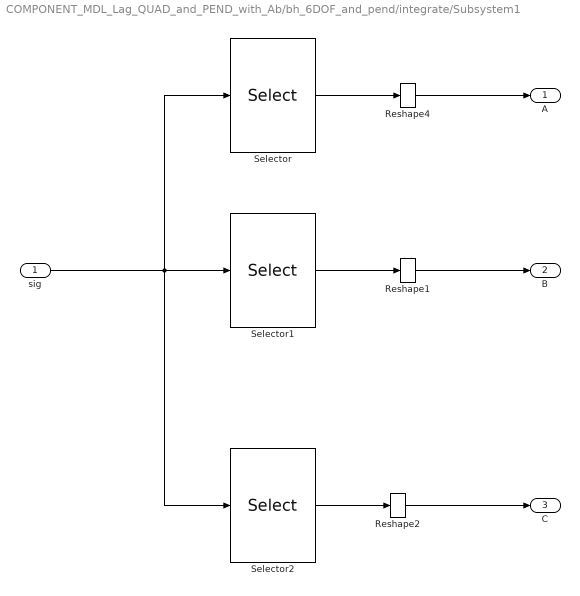
== system COMPONENT_MDL_Lag_QUAD_and_PEND_with_Ab/bh_6DOF_and_pend/integrate/Subsystem1 ==
  sig : Inport
  Reshape1 : Reshape  OutputDimensionality=Column vector (2-D)
  Reshape2 : Reshape  OutputDimensionality=Column vector (2-D)
  Reshape4 : Reshape  OutputDimensionality=Column vector (2-D)
  Selector : Selector  InputPortWidth=9  IndexOptions=Index vector (dialog)  Indices=1:3  OutputSizes=1
  Selector1 : Selector  InputPortWidth=9  IndexOptions=Index vector (dialog)  Indices=4:6  OutputSizes=1
  Selector2 : Selector  InputPortWidth=9  IndexOptions=Index vector (dialog)  Indices=7:9  OutputSizes=1
  A : Outport  VectorParamsAs1DForOutWhenUnconnected=off
  B : Outport  Port=2  VectorParamsAs1DForOutWhenUnconnected=off
  C : Outport  Port=3  VectorParamsAs1DForOutWhenUnconnected=off
  wires:
  Selector/1 -> Reshape4/1
  Selector2/1 -> Reshape2/1
  Selector1/1 -> Reshape1/1
  sig/1 -> Selector/1, Selector2/1, Selector1/1
  Reshape4/1 -> A/1
  Reshape1/1 -> B/1
  Reshape2/1 -> C/1

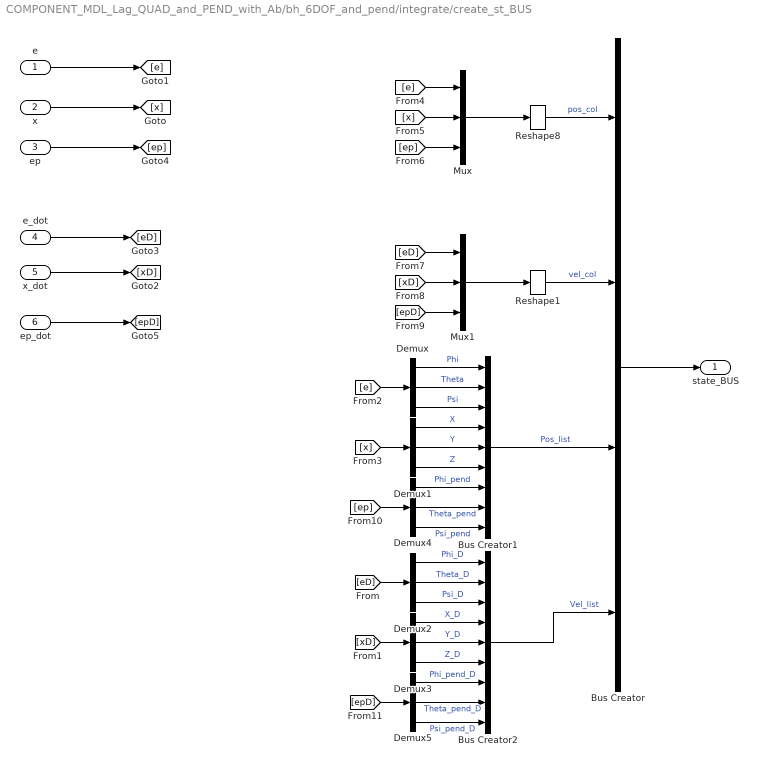
== system COMPONENT_MDL_Lag_QUAD_and_PEND_with_Ab/bh_6DOF_and_pend/integrate/create_st_BUS ==
  e : Inport
  x : Inport  Port=2
  ep : Inport  Port=3
  e_dot : Inport  Port=4
  x_dot : Inport  Port=5
  ep_dot : Inport  Port=6
  Bus Creator : BusCreator  Inputs=4
  Bus Creator1 : BusCreator  Inputs=9
  Bus Creator2 : BusCreator  Inputs=9
  Demux{,1..5} (6 alike) : Demux  Outputs=3
  Mux : Mux  Inputs=3
  Mux1 : Mux  Inputs=3
  Reshape1 : Reshape  OutputDimensionality=Column vector (2-D)
  Reshape8 : Reshape  OutputDimensionality=Column vector (2-D)
  state_BUS : Outport  VectorParamsAs1DForOutWhenUnconnected=off
  wires:
  Mux1/1 -> Reshape1/1
  Mux/1 -> Reshape8/1
  Reshape1/1 -> Bus Creator/2  "vel_col"
  Reshape8/1 -> Bus Creator/1  "pos_col"
  Bus Creator1/1 -> Bus Creator/3  "Pos_list"
  Demux/1 -> Bus Creator1/1  "Phi"
  Demux/2 -> Bus Creator1/2  "Theta"
  Demux/3 -> Bus Creator1/3  "Psi"
  Demux1/2 -> Bus Creator1/5  "Y"
  Demux1/3 -> Bus Creator1/6  "Z"
  Demux1/1 -> Bus Creator1/4  "X"
  [e] -> Demux/1
  [x] -> Demux1/1
  Bus Creator2/1 -> Bus Creator/4  "Vel_list"
  Demux2/1 -> Bus Creator2/1  "Phi_D"
  Demux2/2 -> Bus Creator2/2  "Theta_D"
  Demux2/3 -> Bus Creator2/3  "Psi_D"
  Demux3/1 -> Bus Creator2/4  "X_D"
  Demux3/2 -> Bus Creator2/5  "Y_D"
  Demux3/3 -> Bus Creator2/6  "Z_D"
  [eD] -> Demux2/1
  [xD] -> Demux3/1
  Bus Creator/1 -> state_BUS/1
  ep/1 -> [ep]
  x/1 -> [x]
  e/1 -> [e]
  ep_dot/1 -> [epD]
  x_dot/1 -> [xD]
  e_dot/1 -> [eD]
  [ep] -> Mux/3
  [x] -> Mux/2
  [e] -> Mux/1
  [epD] -> Mux1/3
  [xD] -> Mux1/2
  [eD] -> Mux1/1
  [ep] -> Demux4/1
  Demux4/1 -> Bus Creator1/7  "Phi_pend"
  Demux4/2 -> Bus Creator1/8  "Theta_pend"
  Demux4/3 -> Bus Creator1/9  "Psi_pend"
  [epD] -> Demux5/1
  Demux5/1 -> Bus Creator2/7  "Phi_pend_D"
  Demux5/2 -> Bus Creator2/8  "Theta_pend_D"
  Demux5/3 -> Bus Creator2/9  "Psi_pend_D"

== matlab function COMPONENT_MDL_Lag_QUAD_and_PEND_with_Ab/bh_6DOF_and_pend/Vg_to_Vb/bRg1 ==
  data: phi input; bRg output; theta input; psi input
function bRg = bRg(phi,theta,psi)
%#codegen

%    This function was generated by the Symbolic Math Toolbox version 7.2.
%    28-Aug-2017 09:46:25

bRg = reshape([cos(phi).*cos(theta),-cos(psi).*sin(phi)+cos(phi).*sin(psi).*sin(theta),sin(phi).*sin(psi)+cos(phi).*cos(psi).*sin(theta),cos(theta).*sin(phi),cos(phi).*cos(psi)+sin(phi).*sin(psi).*sin(theta),-cos(phi).*sin(psi)+cos(psi).*sin(phi).*sin(theta),-sin(theta),cos(theta).*sin(psi),cos(psi).*cos(theta)],[3,3]);

== matlab function COMPONENT_MDL_Lag_QUAD_and_PEND_with_Ab/bh_6DOF_and_pend/bRg ==
  data: phi input; bRg output; theta input; psi input
function bRg = bRg(phi,theta,psi)
%#codegen

%    This function was generated by the Symbolic Math Toolbox version 7.2.
%    28-Aug-2017 08:55:21

bRg = reshape([cos(phi).*cos(theta),-cos(psi).*sin(phi)+cos(phi).*sin(psi).*sin(theta),sin(phi).*sin(psi)+cos(phi).*cos(psi).*sin(theta),cos(theta).*sin(phi),cos(phi).*cos(psi)+sin(phi).*sin(psi).*sin(theta),-cos(phi).*sin(psi)+cos(psi).*sin(phi).*sin(theta),-sin(theta),cos(theta).*sin(psi),cos(psi).*cos(theta)],[3,3]);

== matlab function COMPONENT_MDL_Lag_QUAD_and_PEND_with_Ab/bh_6DOF_and_pend/calc_wb/calc_w_from_eul_rates ==
  data: THE_Theta input; wb output; THE_Psi input; THE_PhiD input; THE_ThetaD input; THE_PsiD input
function wb = calc_w_from_eul_rates(THE_Theta,THE_Psi,THE_PhiD,THE_ThetaD,THE_PsiD)
%#codegen

%    This function was generated by the Symbolic Math Toolbox version 7.2.
%    28-Aug-2017 10:05:21

wb = [THE_PsiD-THE_PhiD.*sin(THE_Theta);THE_ThetaD.*cos(THE_Psi)+THE_PhiD.*cos(THE_Theta).*sin(THE_Psi);-THE_ThetaD.*sin(THE_Psi)+THE_PhiD.*cos(THE_Psi).*cos(THE_Theta)];

== matlab function COMPONENT_MDL_Lag_QUAD_and_PEND_with_Ab/bh_6DOF_and_pend/integrate/bRg ==
  data: phi input; bRg output; theta input; psi input
function bRg = bRg(phi,theta,psi)
%#codegen

%    This function was generated by the Symbolic Math Toolbox version 7.2.
%    28-Aug-2017 10:05:16

bRg = reshape([cos(phi).*cos(theta),-cos(psi).*sin(phi)+cos(phi).*sin(psi).*sin(theta),sin(phi).*sin(psi)+cos(phi).*cos(psi).*sin(theta),cos(theta).*sin(phi),cos(phi).*cos(psi)+sin(phi).*sin(psi).*sin(theta),-cos(phi).*sin(psi)+cos(psi).*sin(phi).*sin(theta),-sin(theta),cos(theta).*sin(psi),cos(psi).*cos(theta)],[3,3]);

== matlab function COMPONENT_MDL_Lag_QUAD_and_PEND_with_Ab/bh_6DOF_and_pend/create pend_BUS/MATLAB Function ==
  data: phi input; wb output; theta input; psi input; phi_dot input; theta_dot input; psi_dot input
function wb = fcn(phi,theta,psi, phi_dot, theta_dot, psi_dot)

A = [ ...
             -sin(theta),         0, 1;
        cos(theta)*sin(psi),  cos(psi), 0;
        cos(psi)*cos(theta), -sin(psi), 0;  ];


x = [    phi_dot;
       theta_dot; 
         psi_dot;  ];  
    


wb = A * x;

== matlab function COMPONENT_MDL_Lag_QUAD_and_PEND_with_Ab/bh_6DOF_and_pend/integrate/calc_eul_rates_from_w ==
  data: THE_Theta input; edot output; THE_Psi input; p input; q input; r input
function edot = calc_eul_rates_from_w(THE_Theta,THE_Psi,p,q,r)
%#codegen

%    This function was generated by the Symbolic Math Toolbox version 7.2.
%    28-Aug-2017 10:05:22

edot = [(r.*cos(THE_Psi)+q.*sin(THE_Psi))./cos(THE_Theta);q.*cos(THE_Psi)-r.*sin(THE_Psi);(p.*cos(THE_Theta)+r.*cos(THE_Psi).*sin(THE_Theta)+q.*sin(THE_Psi).*sin(THE_Theta))./cos(THE_Theta)];

== matlab function COMPONENT_MDL_Lag_QUAD_and_PEND_with_Ab/bh_6DOF_and_pend/create pend_BUS/bRg ==
  data: phi input; bRg output; theta input; psi input
function bRg = bRg(phi,theta,psi)
%#codegen

%    This function was generated by the Symbolic Math Toolbox version 7.2.
%    28-Aug-2017 08:55:21

bRg = reshape([cos(phi).*cos(theta),-cos(psi).*sin(phi)+cos(phi).*sin(psi).*sin(theta),sin(phi).*sin(psi)+cos(phi).*cos(psi).*sin(theta),cos(theta).*sin(phi),cos(phi).*cos(psi)+sin(phi).*sin(psi).*sin(theta),-cos(phi).*sin(psi)+cos(psi).*sin(phi).*sin(theta),-sin(theta),cos(theta).*sin(psi),cos(psi).*cos(theta)],[3,3]);

== matlab function COMPONENT_MDL_Lag_QUAD_and_PEND_with_Ab/bh_6DOF_and_pend/MATLAB Function ==
  data: I input; Ixx output; Ixy output; Ixz output; Iyy output; Iyz output; Izz output
function [Ixx, Ixy, Ixz, Iyy, Iyz, Izz] = fcn(I)

Ixx = I(1,1); 
Ixy = I(1,2); 
Ixz = I(1,3); 
Iyy = I(2,2); 
Iyz = I(2,3); 
Izz = I(3,3);

end

== matlab function COMPONENT_MDL_Lag_QUAD_and_PEND_with_Ab/bh_6DOF_and_pend/MATLAB Function1 ==
  data: I input; Ixx output; Ixy output; Ixz output; Iyy output; Iyz output; Izz output
function [Ixx, Ixy, Ixz, Iyy, Iyz, Izz] = fcn(I)

Ixx = I(1,1); 
Ixy = I(1,2); 
Ixz = I(1,3); 
Iyy = I(2,2); 
Iyz = I(2,3); 
Izz = I(3,3);

end
